simulink model "simple_battery_mdl_cycle"  (R2023b)
settings: Solver=VariableStepAuto  StartTime=0.0  StopTime=tend  RelTol=1e-6
values from neighbouring files (symbols this model uses):
  cyc_time = Qo / I * 3600    (= 3600)    [sim_battery_mdl.m]
  I = Qo * C_rate    (= 24)    [sim_battery_mdl.m]
undefined symbols (not defined in the file or in its folder): Ion, Lithium
libraries: spsBatteryLib x1, spsControlledCurrentSourceLib x1, spsTriangleGeneratorLib x1, sps_lib x1
settings Model: Creator=amico44  LastModifiedBy=arvba41

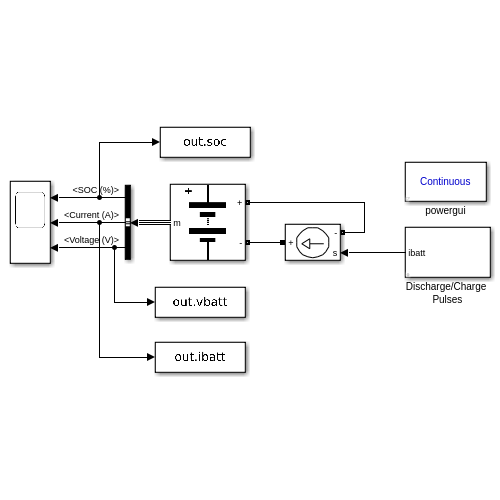
[thumbnail: Simulink's stored preview of the top-level diagram]
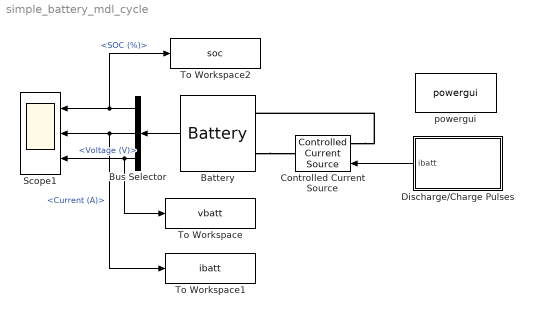
== system simple_battery_mdl_cycle ==
  Battery : spsBatteryLib/Battery  BatType=Lithium-Ion  ShowTempParam=off  ThermalPreset=no  ShowAgeParam=off  NomV=3.58  NomQ=Qo  SOC=Qinit  Batt_Tr=30  PresetModel=on  MaxQ=24  MinV=2.685  FullV=4.1671  Dis_rate=10.4348  R=0.0015  Normal_OP=21.7043  expZone="[3.8678      1.1791]"  current=[6.5 13 32.5]  Units=Ampere-hour  Tci=20  NomT=20  T2=-30  MaxQ2=4.8  FullV2=7.1  Normal_OP2=5.655  expZone2="[6.58           1]"  Rca=0.6  ti=2000  Dp=0  Neq0=0  Tsim=1e6  Ta1=25  Qeol=5.4*0.9  Reol=0.013333*1.2  Char_age=[2.3478, 3]  Dis_age=[2.3478, 10]  N1=1500  N2=10500  N3=1000  N4=1400  Ta2=45  N5=950
  Bus Selector : BusSelector  OutputSignals=SOC (%),Current (A),Voltage (V)
  Controlled Current Source : spsControlledCurrentSourceLib/Controlled Current Source  Initialize=on  Source_Type=AC  Amplitude=0  Phase=0  Frequency=0  Measurements=None
  Discharge/Charge Pulses : Subsystem  mask{In=I, Ip=I}
      mask prompts: In "Charge current [A]"; Ip "Discharge current [A]"
  Scope1 : Scope  NumInputPorts=3
  To Workspace : ToWorkspace  VariableName=vbatt  SampleTime=-1
      settings: Save2DSignal=2-D array (concatenate along first dimension)
  To Workspace1 : ToWorkspace  VariableName=ibatt  SampleTime=-1
      settings: Save2DSignal=2-D array (concatenate along first dimension)
  To Workspace2 : ToWorkspace  VariableName=soc  SampleTime=-1
      settings: Save2DSignal=2-D array (concatenate along first dimension)
  powergui : sps_lib/powergui  Priority=1  SimulationMode=Continuous  SampleTime=50e-6  frequency=60  Iterations=50  frequencyindice=0  Pbase=100e6  ErrMax=1e-4  UnitsV=kV  UnitsW=MW  buscounter=0  FunctionMessages=off  echomessages=off  EnableUseOfTLC=off  CurrentSourceSwitches=off  DisableSnubberDevices=off  DisableRonSwitches=off  DisableVfSwitches=off  DisplayEquations=off  AutomaticDiscreteSolvers=off  SolverType=Tustin/Backward Euler (TBE)  Interpol=off  ExternalGateDelay=off  methode=off  Ts=100  x0status=blocks  SPID=on  SwTol=0  HookPort=off  NonlinearTolerance=1e-4  nMaxIteration=100  ContinueOnMaxIteration=off  RestoreLinks=warning  ResistiveCurrentMeasurement=off  Frange=[0:2:500]  Ylog=off  Xlog=on  ShowGrid=off  save=off  variable=ZData  structure=0  ZoomFFT=off  StartTime=0.0  cycles=1  DisplayStyle=1  fundamental=60  FreqAxis=off  MaxFrequency=1000  frequencyindicesteady=1  RmsSteady=1  display=off
  wires:
  Battery/1 -> Bus Selector/1
  Bus Selector/1 -> To Workspace2/1, Scope1/1  "<SOC (%)>"
  Bus Selector/2 -> To Workspace1/1, Scope1/2  "<Current (A)>"
  Bus Selector/3 -> To Workspace/1, Scope1/3  "<Voltage (V)>"
  Discharge/Charge Pulses/1(ibatt) -> Controlled Current Source/1
  connections:
  Controlled Current Source/LConn1 -- Battery/LConn1
  Battery/LConn2 -- Controlled Current Source/RConn1

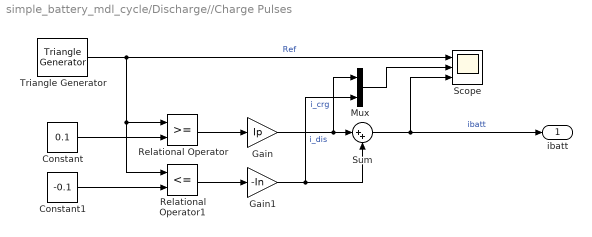
== system simple_battery_mdl_cycle/Discharge//Charge Pulses ==
  Constant : Constant  Value=0.1
  Constant1 : Constant  Value=-0.1
  Gain : Gain  Gain=Ip  ParamDataTypeStr=double
  Gain1 : Gain  Gain=-In  ParamDataTypeStr=double
  Mux : Mux  Inputs=2
  Relational Operator : RelationalOperator  OutDataTypeStr=boolean  RndMeth=Simplest  InputSameDT=off
  Relational Operator1 : RelationalOperator  Operator=<=  OutDataTypeStr=boolean  RndMeth=Simplest  InputSameDT=off
  Scope : Scope  NumInputPorts=3
  Sum : Sum  Inputs=|++
  Triangle Generator : spsTriangleGeneratorLib/Triangle Generator  Freq=1/cyc_time  Phase=90  Ts=0
  ibatt : Outport
  wires:
  Triangle Generator/1 -> Relational Operator/1, Relational Operator1/1, Scope/1  "Ref"
  Mux/1 -> Scope/2
  Constant/1 -> Relational Operator/2
  Sum/1 -> ibatt/1, Scope/3  "ibatt"
  Gain/1 -> Sum/1, Mux/1  "i_crg"
  Gain1/1 -> Sum/2, Mux/2  "i_dis"
  Relational Operator1/1 -> Gain1/1
  Relational Operator/1 -> Gain/1
  Constant1/1 -> Relational Operator1/2
